simulink model "control_model"  (R2018b)
settings: Solver=VariableStepAuto  StartTime=0.0  StopTime=10.0  RelTol=1e-3
libraries: fuzblock x1
settings Model: Creator=student  LastModifiedBy=student

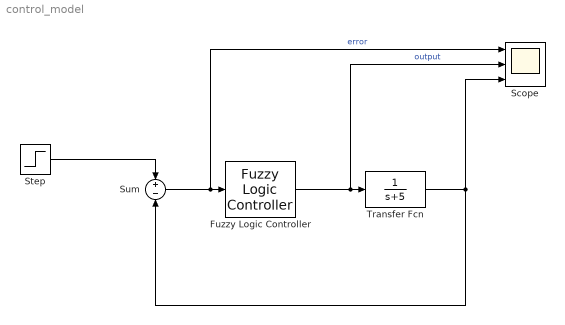
== system control_model ==
  Fuzzy Logic Controller : fuzblock/Fuzzy Logic  Controller  FIS='control.fis'  OutputSampleNumber=101  DataType=double  FuzzifiedInputs=off  RuleFiringStrengths=off  RuleOutputs=off  AggregatedOutputs=off  SimulateUsing=Interpreted execution  OutOfRangeInputValueMessage=warning  NoRuleFiredMessage=warning  EmptyOutputFuzzySetMessage=warning
  Scope : Scope  NumInputPorts=3
  Step : Step  Time=10  SampleTime=0
  Sum : Sum  Inputs=+-
  Transfer Fcn : TransferFcn  Denominator=[1 5]
  wires:
  Fuzzy Logic Controller/1 -> Scope/2, Transfer Fcn/1  "output"
  Sum/1 -> Scope/1, Fuzzy Logic Controller/1  "error"
  Step/1 -> Sum/1
  Transfer Fcn/1 -> Scope/3, Sum/2
